simulink model "MagnetometerProcessing_lib_test"  (R2018b)
settings: Solver=VariableStepAuto  StartTime=0.0  StopTime=1  RelTol=1e-3
libraries: MagnetometerProcessing_lib x1
settings Model: Creator=Nick's PC  LastModifiedBy=Nick's PC

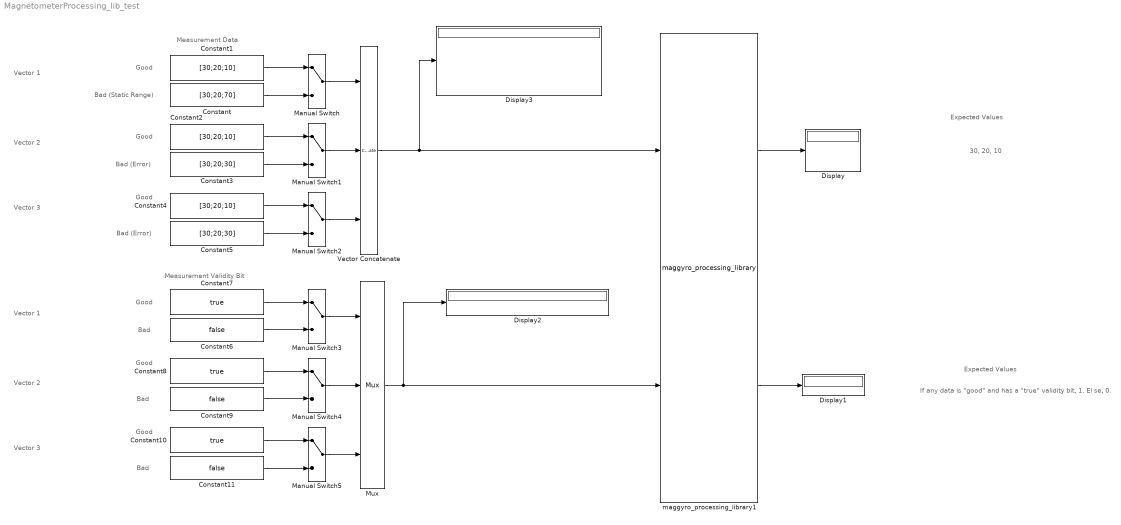
== system MagnetometerProcessing_lib_test ==
  note: Measurement Data
  note: Vector 1
  note: 30, 20, 10
  note: If any data is "good" and has a "true" validity bit, 1. El se, 0.
  note: Expected Values
  note: Bad (Static Range)
  note: Good
  note: Good
  note: Good
  note: Bad (Error)
  note: Bad
  note: Bad
  note: Bad
  note: Good
  note: Good
  note: Good
  note: Bad (Error)
  note: Expected Values
  note: Vector 2
  note: Vector 3
  note: Vector 2
  note: Vector 1
  note: Vector 3
  note: Measurement Validity Bit
  Constant : Constant  Value=[30;20;70]
  Constant1 : Constant  Value=[30;20;10]
  Constant10 : Constant  Value=true
  Constant11 : Constant  Value=false
  Constant2 : Constant  Value=[30;20;10]
  Constant3 : Constant  Value=[30;20;30]
  Constant4 : Constant  Value=[30;20;10]
  Constant5 : Constant  Value=[30;20;30]
  Constant6 : Constant  Value=false
  Constant7 : Constant  Value=true  OutDataTypeStr=boolean
  Constant8 : Constant  Value=true
  Constant9 : Constant  Value=false
  Display{,1..3} (4 alike) : Display
  Manual Switch{,1..5} (6 alike) : ManualSwitch
  Mux : Mux  Inputs=3
  Vector Concatenate : Concatenate  NumInputs=3  Mode=Multidimensional array  ConcatenateDimension=2
  maggyro_processing_library1 : MagnetometerProcessing_lib/maggyro_processing_library  static_range_max_value=fswParams.sensors.mag_static_range  rotation_calibration_matrix1=fswParams.sensors.mag_rotate1  rotation_calibration_matrix2=fswParams.sensors.mag_rotate2  rotation_calibration_matrix3=fswParams.sensors.mag_rotate3  offset_calibration_matrix=fswParams.sensors.mag_offset  mag_max_err=fswParams.sensors.mag_max_err
  wires:
  maggyro_processing_library1/2 -> Display1/1
  maggyro_processing_library1/1 -> Display/1
  Constant1/1 -> Manual Switch/1
  Constant/1 -> Manual Switch/2
  Constant2/1 -> Manual Switch1/1
  Constant3/1 -> Manual Switch1/2
  Constant4/1 -> Manual Switch2/1
  Constant5/1 -> Manual Switch2/2
  Manual Switch1/1 -> Vector Concatenate/2
  Manual Switch/1 -> Vector Concatenate/1
  Manual Switch2/1 -> Vector Concatenate/3
  Vector Concatenate/1 -> maggyro_processing_library1/1, Display3/1
  Manual Switch5/1 -> Mux/3
  Constant10/1 -> Manual Switch5/1
  Mux/1 -> maggyro_processing_library1/2, Display2/1
  Constant7/1 -> Manual Switch3/1
  Constant6/1 -> Manual Switch3/2
  Constant11/1 -> Manual Switch5/2
  Manual Switch4/1 -> Mux/2
  Constant8/1 -> Manual Switch4/1
  Constant9/1 -> Manual Switch4/2
  Manual Switch3/1 -> Mux/1
